simulink model "NEW_MAIN_noDD"  (R2017b)
settings: Solver=ode15s  StartTime=0.0  StopTime=10.0  RelTol=1e-3
values from neighbouring files (symbols this model uses):
  A = eye(16,16)    [full_input_list.m]
  B = zeros(16,1)    [full_input_list.m]
  C = blkdiag(eye(3,3),zeros(3,3),eye(10,10))    [full_input_list.m]
  currentMax_B = [0;0.8;0.2]    [full_input_list.m]
  deltaT = 0.00001    (= 1e-05)    [full_input_list.m]
  epsilon_UD_slew = .01    (= 0.01)    [full_input_list.m]
  epsilon_UD_spinUp = .01    (= 0.01)    [full_input_list.m]
  freq = 80    [full_input_list.m]    (also in initSimulink.m)
  H = C    [full_input_list.m]
  I_UD = [0.032808359, 0.000617048, 0.000049185;      0.000617048, 0.032531573, 0.000060042;      0.000049185, 0.000060042, 0.007799591]    [full_input_list.m]
  kd = 0.5    [full_input_list.m]    (also in initACS.m = 0.01)
  kd_UD_detumble = 6e-3    (= 0.006)    [full_input_list.m]
  kp = 1    [full_input_list.m]    (also in initACS.m = 0.01)
  magMomentMax_B = sat2CoilArea.*sat2n.*currentMax_B    [full_input_list.m]
  omega_cmd_N = 1e-1*[1 1 -.6]'    [full_input_list.m]
  omega_spinUp_MAG = 0.05    [full_input_list.m]
  OpModes = [0 0 0]    [full_input_list.m]
  OpTimes = [0 1 2]    [full_input_list.m]
  q4_cmd_init = [q4_cmd_init(2:4); q4_cmd_init(1)]    [full_input_list.m]
  Q_k = zeros(16,16)    [full_input_list.m]
  R = R_k    [full_input_list.m]
  sat2CoilArea = 0.8*[0.02; 0.02; 0.01]    [full_input_list.m]
  sat2n = [0; 100; 100]    [full_input_list.m]
  sat2Resistance = sat2WireLength.*sat2WireResistivity./sat2WireArea    [full_input_list.m]
  SeperationTime = 30000    [full_input_list.m]
  spinAxis_B = [1 0 0]    [full_input_list.m]
  u_k = zeros(16,1)    [full_input_list.m]
  w_k = zeros(16,1)    [full_input_list.m]
  Z_k = zeros(16,1)    [full_input_list.m]
undefined symbols (not defined in the file or in its folder): B_n, B_N, DiscIntNeverNeededParam, G_igrf, gyro_DCM_BS, H_igrf, I_B, IAU, Kschmidt, mag_variance, Orbit_time, R_mean, r_n, r_N, v_n, v_N
libraries: aerolibutil x53, vrlib x37, simulink x22, SimMainLibrary x14, dspmathops x6, sharedtransform x4, dspinverses x2, dspmtrx3 x1, aerolibtransform2 x1, aerolibgravity2 x1, lib_violet_env x1
(part 1 of 3)
settings Model: Creator=vtroo  LastModifiedBy=vtroo

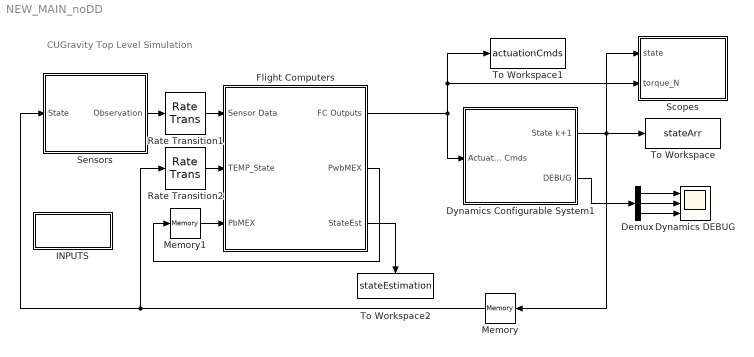
== system NEW_MAIN_noDD ==
  note: CUGravity Top Level Simulation
  Demux : Demux  Outputs=3
  Dynamics Configurable System1 : Subsystem  BlockChoice=Three Link Simscape Model
      link override Extendable Single  Link Simscape /s_teth_init2: PxPositionTargetSpecify=on  PxPositionTargetValue=eps
      link override Single Link Simscape Model/s_teth_init: PxPositionTargetSpecify=on  PxPositionTargetValue=eps  PyPositionTargetSpecify=on  PyPositionTargetValue=eps  PzPositionTargetSpecify=on  PzPositionTargetValue=eps
      link override Single Link Simscape Model/s_teth_init2: PxPositionTargetSpecify=on  PxPositionTargetValue=eps  PyPositionTargetSpecify=on  PyPositionTargetValue=eps  PzPositionTargetSpecify=on  PzPositionTargetValue=eps
      link override Three Link Simscape Model/Attitude Disturbance Model/Aerodynamic Drag/Constant1: Value=G*m_earth
      link override Three Link Simscape Model/Attitude Disturbance Model/Aerodynamic Drag/Gain: Gain=0.5*cd*Ab*p
      link override Three Link Simscape Model/Attitude Disturbance Model/Gravity Gradient/X-Torque/Constant: Value=3*G*m_earth*(I3-I2)
      link override Three Link Simscape Model/Attitude Disturbance Model/Gravity Gradient/Y-Torque/Constant: Value=3*G*m_earth*(I1-I3)
      link override Three Link Simscape Model/Attitude Disturbance Model/Gravity Gradient/Z-Torque/Constant: Value=3*G*m_earth*(I2-I1)
      link override Three Link Simscape Model/Attitude Disturbance Model/Solar Radiation Pressure/Gain: Gain=(flux/c)*Ab*(1+q)
      link override Three Link Simscape Model/Attitude Disturbance Model/Solar Radiation Pressure/Gain1: Gain=(flux/c)*Ab*(1+q)
      link override Three Link Simscape Model/Attitude Disturbance Model/Solar Radiation Pressure/Gain2: Gain=(flux/c)*Ab*(1+q)
      link override Three Link Simscape Model/Bus Selector1: OutputSignals=CenterCube_PWM_cmds,MotorReelRates,BurnCmd,ACSSafeMode
      link override Three Link Simscape Model/CenterSat_6DOF: PxVelocityTargetPriority=Low  PyVelocityTargetPriority=Low  PzVelocityTargetPriority=Low
      link override Three Link Simscape Model/EndSat1_6DOF: PxVelocityTargetPriority=Low  PyVelocityTargetPriority=Low  PzVelocityTargetPriority=Low
      link override Three Link Simscape Model/EndSat2_6DOF: PxVelocityTargetPriority=Low  PyVelocityTargetPriority=Low  PzVelocityTargetPriority=Low
      link override Three Link Simscape Model/Kane Damper 1: SerializedFrames=<Frames><Frame><Id>Frame1</Id><Value><Name>F1</Name><Origin><Source>GeometricFeature</Source><FeatureName>+z surface</FeatureName></Origin><PrimaryAxis><DefinedDirection>+Z</DefinedDirection><Source>ReferenceFrame</Source><SourceDirection>+Z</SourceDirection><FeatureName></FeatureName></PrimaryAxis><SecondaryAxis><DefinedDirection>+X</DefinedDirection><Source>ReferenceFrame</Source><SourceDirection>+X</SourceDirection><FeatureName></FeatureName></SecondaryAxis></Value></Frame></Frames>
      link override Three Link Simscape Model/Kane Damper 2: SerializedFrames=<Frames><Frame><Id>Frame1</Id><Value><Name>F1</Name><Origin><Source>GeometricFeature</Source><FeatureName>-z surface</FeatureName></Origin><PrimaryAxis><DefinedDirection>+Z</DefinedDirection><Source>ReferenceFrame</Source><SourceDirection>+Z</SourceDirection><FeatureName></FeatureName></PrimaryAxis><SecondaryAxis><DefinedDirection>+X</DefinedDirection><Source>ReferenceFrame</Source><SourceDirection>+X</SourceDirection><FeatureName></FeatureName></SecondaryAxis></Value></Frame></Frames>  GeometryShape=Brick  BrickDimensions=[kane_radius kane_radius kane_height]
      link override Three Link Simscape Model/Linear Damper: SpringStiffness=1/(1/linearDamper_k + 1/((pi*teth_radius_actual^2)*teth_modulus/teth_length))
      link override Undeployed Model/Center Sat1: GraphicDiffuseColor=[0.0 0.8 0.8]  GraphicOpacity=.5  SerializedFrames=<Frames><Frame><Id>Frame1</Id><Value><Name>PosZ</Name><Origin><Source>GeometricFeature</Source><FeatureName>+z surface</FeatureName></Origin><PrimaryAxis><DefinedDirection>+Z</DefinedDirection><Source>ReferenceFrame</Source><SourceDirection>+Z</SourceDirection><FeatureName></FeatureName></PrimaryAxis><SecondaryAxis><DefinedDirection>+X</DefinedDirection><Source>ReferenceFrame</Source><SourceDirection>+X</SourceDirection><FeatureName></FeatureName></SecondaryAxis></Value></Frame><Frame><Id>Frame2</Id><Value><Name>NegZ</Name><Origin><Source>GeometricFeature</Source><FeatureName>-z surface</FeatureName></Origin><PrimaryAxis><DefinedDirection>+Z</DefinedDirection><Source>ReferenceFrame</Source><SourceDirection>+Z</SourceDirection><FeatureName></FeatureName></PrimaryAxis><SecondaryAxis><DefinedDirection>+X</DefinedDirection><Source>ReferenceFrame</Source><SourceDirection>+X</SourceDirection><FeatureName></FeatureName></SecondaryAxis></Value></Frame><Frame><Id>Frame7</Id><Value><Name>PosX</Name><Origin><Source>GeometricFeature</Source><FeatureName>+x surface</FeatureName></Origin><PrimaryAxis><DefinedDirection>+Z</DefinedDirection><Source>ReferenceFrame</Source><SourceDirection>+Z</SourceDirection><FeatureName></FeatureName></PrimaryAxis><SecondaryAxis><DefinedDirection>+X</DefinedDirection><Source>ReferenceFrame</Source><SourceDirection>+X</SourceDirection><FeatureName></FeatureName></SecondaryAxis></Value></Frame><Frame><Id>Frame8</Id><Value><Name>COM</Name><Origin><Source>CenterOfMassFrame</Source><FeatureName></FeatureName></Origin><PrimaryAxis><DefinedDirection>+Z</DefinedDirection><Source>ReferenceFrame</Source><SourceDirection>+Z</SourceDirection><FeatureName></FeatureName></PrimaryAxis><SecondaryAxis><DefinedDirection>+X</DefinedDirection><Source>ReferenceFrame</Source><SourceDirection>+X</SourceDirection><FeatureName></FeatureName></SecondaryAxis></Value></Frame></Frames>
      link override Undeployed Model/EndSat3: GraphicOpacity=.5  GraphicDiffuseColor=[1.0 0.0 0.0]
      link override Undeployed Model/EndSat4: GraphicOpacity=.5  GraphicDiffuseColor=[1.0 0.0 0.0]
      settings: AttributesFormatString=%<BlockChoice>  TemplateBlock=SimMainLibrary/Dynamics Configurable System  MemberBlocks="Extendable Single  Link Simscape ,Single Link Simscape Model,Three Link Simscape Model,Undeployed Model"
  Dynamics DEBUG : Scope  NumInputPorts=3
  Flight Computers : Subsystem  mask(Flight Computers){}
      mask help:
      | The flight computers read in the measured state from the sensor block and the previous PowerBoard commands and state (inputs). The ground commands are also inputs to receive potential command override. This information is then passed through the Kalman filter to estimate the state and remove sensor noise, and sent through a controller which determines the operation mode, updated PowerBoard Status, and actuator commands. These outputs govern the operation of the satellite and deterine the trajectory it will follow in the future steps.
      |
      | NOTE: Currently the UKF is not complete, and for that reason the input state read into the controller is simply the exact state outputted from the dynamics block. That is, the sensor block is going unused because there is no way to currently remove sensor noise (UKF). Once the UKF is completed, the sensor measurements must be used for the controller inputs to simulate a more realistic environment.
  INPUTS : Subsystem
  Memory : Memory  InheritSampleTime=on
  Memory1 : Memory  InheritSampleTime=on
  Rate Transition1 : RateTransition  OutPortSampleTime=1/freq
  Rate Transition2 : RateTransition  OutPortSampleTime=1/freq
  Scopes : Subsystem
  Sensors : Subsystem  mask(State Estimation){}
      mask help:
      | Current Function:
      | This block uses the plant model calculated state (input) and adds sensor noise to the system to calculate the estimated state (output) that is measured and fed into the flight computer. The middle satellite has a more extensive set of calculations required to complete the state estimation, than do the end satellites. All three satellites compute the accelerometer, magnetometer, angular velocity, and sun sensor vector measurements. The middle satellite performs additional calculations to accurately measure simulation time and inertial position of the center of mass.
      |
      | Future Tasks:
      | 1. Make sure that q1_BN is quaternion of B relative to N, otherwise rotation may be in the wrong direction.
      | 2. Need to test the calculation to find the sun vector in the B frame.
  To Workspace : ToWorkspace  VariableName=stateArr  SaveFormat=Timeseries  SampleTime=-1
  To Workspace1 : ToWorkspace  VariableName=actuationCmds  SaveFormat=Timeseries  SampleTime=-1
  To Workspace2 : ToWorkspace  VariableName=stateEstimation  SaveFormat=Timeseries  SampleTime=-1
  wires:
  Rate Transition1/1 -> Flight Computers/1(Sensor Data)
  Flight Computers/1(FC Outputs) -> To Workspace1/1, Scopes/2(torque_N), Dynamics Configurable System1/1(Actuation Cmds)
  Demux/3 -> Dynamics DEBUG/3
  Rate Transition2/1 -> Flight Computers/2(TEMP_State)
  Demux/2 -> Dynamics DEBUG/2
  Flight Computers/2(PwbMEX) -> Memory1/1
  Dynamics Configurable System1/1(State k+1) -> Scopes/1(state), Memory/1, To Workspace/1
  Sensors/1(Observation) -> Rate Transition1/1
  Flight Computers/3(StateEst) -> To Workspace2/1
  Demux/1 -> Dynamics DEBUG/1
  Memory/1 -> Sensors/1(State), Rate Transition2/1
  Memory1/1 -> Flight Computers/3(PbMEX)
  Dynamics Configurable System1/2(DEBUG) -> Demux/1

== system NEW_MAIN_noDD/Dynamics Configurable System1 ==
  Actuation Cmds : Inport
  Three Link Simscape Model : SimMainLibrary/Three Link Simscape Model
      settings: SourceProductName=CUGravity Library
  State k+1 : Outport
  DEBUG : Outport  Port=2
  wires:
  Actuation Cmds/1 -> Three Link Simscape Model/1
  Three Link Simscape Model/1 -> State k+1/1
  Three Link Simscape Model/2 -> DEBUG/1

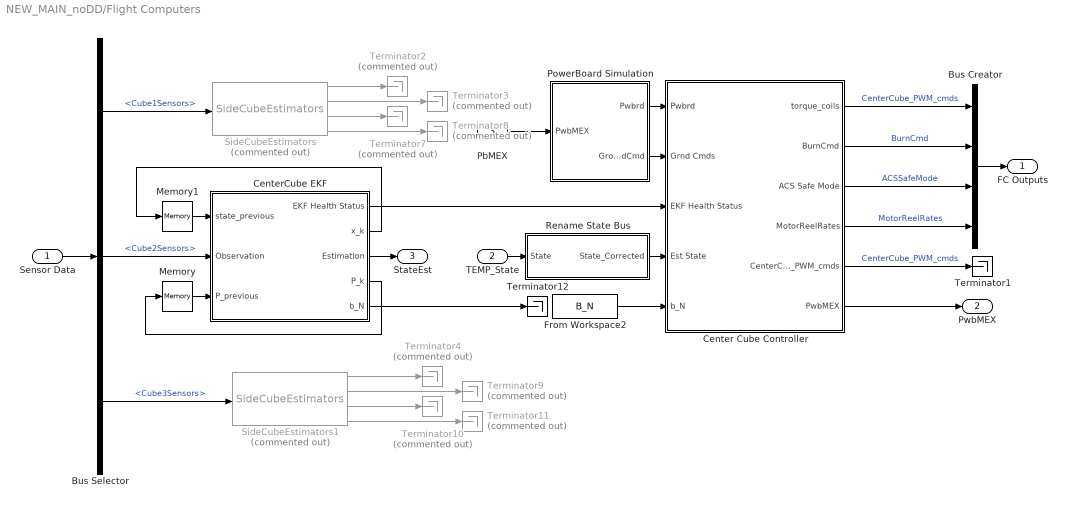
== system NEW_MAIN_noDD/Flight Computers ==
  Sensor Data : Inport
  TEMP_State : Inport  Port=2
  PbMEX : Inport  Port=3
  Bus Creator : BusCreator  Inputs=4
  Bus Selector : BusSelector  OutputSignals=Cube1Sensors,Cube2Sensors,Cube3Sensors
  Center Cube Controller : Subsystem
  CenterCube EKF : Subsystem
  From Workspace2 : FromWorkspace  VariableName=B_N  SampleTime=1/freq
  Memory : Memory
  Memory1 : Memory
  PowerBoard Simulation : Subsystem  mask(Command and Operation){}
      mask help:
      | Current Function:
      | Determines commands based on the PowerBoard as well as messages received from ground control. It also has the status of the sensor and torque actuator signals to feed into the state machine.
      |
      | Future Tasks:
      | Currently the ground commands and PowerBoard commands are the same, so there should probably be a way to allow manual override for ground control purposes.
  Rename State Bus : Subsystem  mask(State Correction){}
      mask help:
      | Current Function:
      | This block is only a PLACEHOLDER for the time being: until the UKF is complete, this block shall be used to feed in the EXACT state (dynamics) to the controller. However, the memory block causes issues with the initial condition for the quaternions, so this block performs a correction such that the norm of the quaternion is always unity (one). Additionally, the connections within the bus must be named as estimated values to be compatible with calculations performed within the controller.
      |
      | Future Task:
      | Complete UKF. Delete this subsystem. Feed the Estimated state output from the UKF into the controller (instead of this output).
  SideCubeEstimators : SimMainLibrary/SideCubeEstimators  Commented=on
      settings: SourceProductName=CUGravity Library
  SideCubeEstimators1 : SimMainLibrary/SideCubeEstimators  Commented=on
      settings: SourceProductName=CUGravity Library
  Terminator1 : Terminator
  Terminator{2..4,7..11} (8 alike) : Terminator  Commented=on
  Terminator12 : Terminator
  FC Outputs : Outport
  PwbMEX : Outport  Port=2
  StateEst : Outport  Port=3
  wires:
  Sensor Data/1 -> Bus Selector/1
  Bus Selector/1 -> SideCubeEstimators/1  "<Cube1Sensors>"
  Bus Selector/2 -> CenterCube EKF/2(Observation)  "<Cube2Sensors>"
  Bus Selector/3 -> SideCubeEstimators1/1  "<Cube3Sensors>"
  SideCubeEstimators/1 -> Terminator2/1
  Bus Creator/1 -> FC Outputs/1
  Center Cube Controller/2(BurnCmd) -> Bus Creator/2  "BurnCmd"
  CenterCube EKF/1(EKF Health Status) -> Center Cube Controller/3("EKF Health Status ")
  Center Cube Controller/6(PwbMEX) -> PwbMEX/1
  CenterCube EKF/3(Estimation) -> StateEst/1
  Center Cube Controller/5(CenterCube_PWM_cmds) -> Terminator1/1  "CenterCube_PWM_cmds"
  SideCubeEstimators/2 -> Terminator3/1
  CenterCube EKF/2(x_k) -> Memory1/1
  CenterCube EKF/4(P_k) -> Memory/1
  SideCubeEstimators/3 -> Terminator7/1
  SideCubeEstimators/4 -> Terminator8/1
  SideCubeEstimators1/1 -> Terminator4/1
  SideCubeEstimators1/2 -> Terminator9/1
  SideCubeEstimators1/3 -> Terminator10/1
  SideCubeEstimators1/4 -> Terminator11/1
  Center Cube Controller/3(ACS Safe Mode) -> Bus Creator/3  "ACSSafeMode"
  Center Cube Controller/4(MotorReelRates) -> Bus Creator/4  "MotorReelRates"
  Center Cube Controller/1(torque_coils) -> Bus Creator/1  "CenterCube_PWM_cmds"
  From Workspace2/1 -> Center Cube Controller/5(b_N)
  CenterCube EKF/5(b_N) -> Terminator12/1
  TEMP_State/1 -> Rename State Bus/1(State)
  PbMEX/1 -> PowerBoard Simulation/1(PwbMEX)
  PowerBoard Simulation/1(Pwbrd) -> Center Cube Controller/1(Pwbrd)
  PowerBoard Simulation/2(GroundCmd) -> Center Cube Controller/2(Grnd Cmds)
  Rename State Bus/1(State_Corrected) -> Center Cube Controller/4(Est State)
  Memory/1 -> CenterCube EKF/3(P_previous)
  Memory1/1 -> CenterCube EKF/1(state_previous)

== system NEW_MAIN_noDD/INPUTS ==
  Chart : Stateflow chart  Commented=on  TreatAsAtomicUnit=on
  Clock : Clock  Commented=on
  Constant : Constant  Commented=on  Value=Orbit_time
  Constant1 : Constant  Commented=on  Value=r_n
  Constant2 : Constant  Commented=on  Value=v_n
  Constant3 : Constant  Commented=on  Value=B_n
  Constant4 : Constant  Commented=on  Value=Orbit_time(1)
  Constant5 : Constant  Commented=on  Value=ones(1,length(Orbit_time))
  Constant6 : Constant  Commented=on  Value=r_N
  Constant7 : Constant  Commented=on  Value=v_N
  Constant8 : Constant  Commented=on  Value=B_N
  From Workspace : FromWorkspace  Commented=on  VariableName=r_N  SampleTime=1/freq
  From Workspace1 : FromWorkspace  Commented=on  VariableName=v_N  SampleTime=1/freq
  From Workspace2 : FromWorkspace  Commented=on  VariableName=B_N  SampleTime=1/freq
  Product : Product  Commented=on
  Sum : Sum  Commented=on  Inputs=|+-
  Terminator : Terminator  Commented=on
  Terminator1 : Terminator  Commented=on
  Terminator2 : Terminator  Commented=on
  wires:
  Clock/1 -> Product/2
  Constant/1 -> Sum/1
  Constant1/1 -> Chart/3(r_N)
  Constant2/1 -> Chart/4(v_N)
  Constant3/1 -> Chart/5(B_N)
  Sum/1 -> Chart/2(T)
  Constant4/1 -> Sum/2
  Product/1 -> Chart/1(t)
  Constant5/1 -> Product/1
  Chart/1(r) -> Terminator/1
  Chart/2(v) -> Terminator1/1
  Chart/3(B) -> Terminator2/1

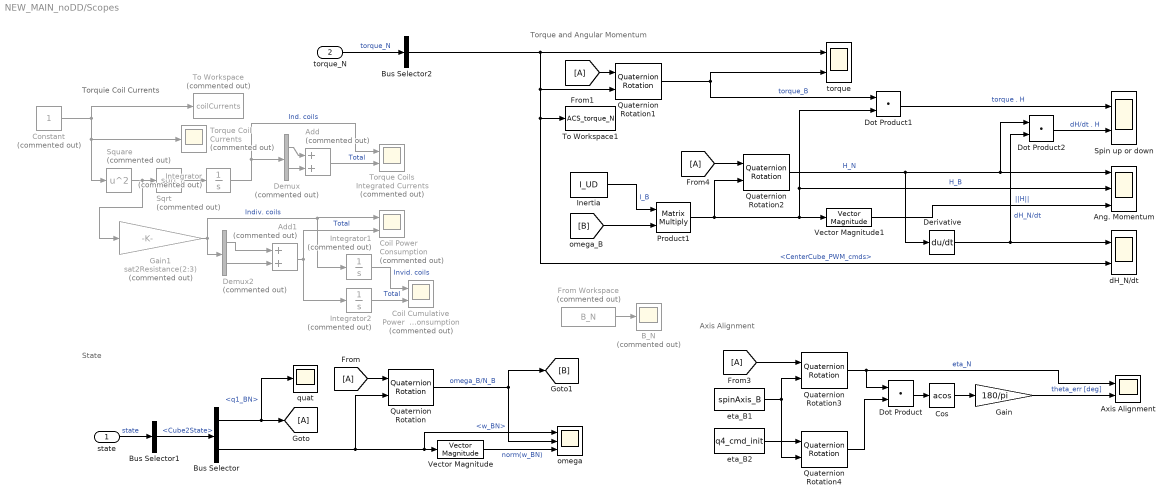
== system NEW_MAIN_noDD/Scopes ==
  note: State
  note: Torque and Angular Momentum
  note: Axis Alignment
  note: Torquie Coil Currents
  state : Inport
  torque_N : Inport  Port=2
  Add : Sum  Commented=on
  Add1 : Sum  Commented=on
  Ang. Momentum : Scope  NumInputPorts=3
  Axis Alignment : Scope  NumInputPorts=2
  B_N : Scope  Commented=on
  Bus Selector : BusSelector  OutputSignals=q1_BN,w_BN
  Bus Selector1 : BusSelector  OutputSignals=Cube2State
  Bus Selector2 : BusSelector  OutputSignals=CenterCube_PWM_cmds
  Coil Cumulative Power  Consumption : Scope  Commented=on  NumInputPorts=2
  Coil Power Consumption : Scope  Commented=on  NumInputPorts=2
  Constant : Constant  Commented=on
  Cos : Trigonometry  Operator=acos  OutputSignalType=real
  Demux : Demux  Commented=on  Outputs=2
  Demux2 : Demux  Commented=on  Outputs=2
  Derivative : Derivative
  Dot Product : DotProduct  InputSameDT=on  OutDataTypeStr=Inherit: Inherit via internal rule
  Dot Product1 : DotProduct  InputSameDT=on  OutDataTypeStr=Inherit: Inherit via internal rule
  Dot Product2 : DotProduct  InputSameDT=on  OutDataTypeStr=Inherit: Inherit via internal rule
  From Workspace : FromWorkspace  Commented=on  VariableName=B_N  SampleTime=0
  Gain : Gain  Gain=180/pi
  Gain1 : Gain  Commented=on  Gain=sat2Resistance(2:3)
  Inertia : Constant  Value=I_UD
  Integrator : Integrator  Commented=on
  Integrator1 : Integrator  Commented=on
  Integrator2 : Integrator  Commented=on
  Product1 : Product  Multiplication=Matrix(*)
  Quaternion Rotation{,1..4} (5 alike) : aerolibutil/Quaternion Rotation
  Spin up or down : Scope  NumInputPorts=2
  Sqrt : Sqrt  Commented=on  SaturateOnIntegerOverflow=on
  Square : Math  Commented=on  Operator=square  RndMeth=Zero  SaturateOnIntegerOverflow=on
  To Workspace : ToWorkspace  Commented=on  VariableName=coilCurrents  SaveFormat=Timeseries  SampleTime=-1
  To Workspace1 : ToWorkspace  VariableName=ACS_torque_N  SaveFormat=Timeseries  SampleTime=-1
  Torque Coil Currents : Scope  Commented=on
  Torque Coils Integrated Currents : Scope  Commented=on  NumInputPorts=2
  Vector Magnitude : SimMainLibrary/Vector Magnitude
      settings: SourceProductName=CUGravity Library
  Vector Magnitude1 : SimMainLibrary/Vector Magnitude
      settings: SourceProductName=CUGravity Library
  dH_N/dt : Scope  NumInputPorts=2
  eta_B1 : Constant  Value=spinAxis_B
  eta_B2 : Constant  Value=q4_cmd_init
  omega : Scope  NumInputPorts=3
  quat : Scope
  torque : Scope  NumInputPorts=2
  wires:
  Constant/1 -> Square/1, Torque Coil Currents/1, To Workspace/1
  Integrator/1 -> Demux/1, Torque Coils Integrated Currents/1  "Ind. coils"
  Cos/1 -> Gain/1
  Quaternion Rotation3/1 -> Dot Product/1, Axis Alignment/1  "eta_N"
  eta_B1/1 -> Quaternion Rotation4/2, Quaternion Rotation3/2
  Quaternion Rotation4/1 -> Dot Product/2
  eta_B2/1 -> Quaternion Rotation4/1
  [A] -> Quaternion Rotation3/1
  Dot Product/1 -> Cos/1
  Gain/1 -> Axis Alignment/2  "theta_err [deg]"
  Bus Selector2/1 -> dH_N/dt/2, To Workspace1/1, Quaternion Rotation1/2, torque/1  "<CenterCube_PWM_cmds>"
  [B] -> Product1/2
  Dot Product1/1 -> Spin up or down/1  "torque . H"
  Derivative/1 -> Dot Product2/2, dH_N/dt/1  "dH_N/dt"
  Vector Magnitude1/1 -> Ang. Momentum/3  "||H||"
  [A] -> Quaternion Rotation1/1
  Product1/1 -> Vector Magnitude1/1, Ang. Momentum/2, Dot Product1/2, Quaternion Rotation2/2  "H_B"
  Inertia/1 -> Product1/1  "I_B"
  Quaternion Rotation1/1 -> Dot Product1/1, torque/2  "torque_B"
  [A] -> Quaternion Rotation2/1
  Quaternion Rotation2/1 -> Derivative/1, Dot Product2/1, Ang. Momentum/1  "H_N"
  Bus Selector/2 -> Quaternion Rotation/2, omega/1, Vector Magnitude/1  "<w_BN>"
  Quaternion Rotation/1 -> omega/2, [B]  "omega_B/N_B"
  Bus Selector/1 -> quat/1, [A]  "<q1_BN>"
  Vector Magnitude/1 -> omega/3  "norm(w_BN)"
  Square/1 -> Gain1/1, Sqrt/1
  Sqrt/1 -> Integrator/1
  Demux/1 -> Add/1
  Demux/2 -> Add/2
  Add/1 -> Torque Coils Integrated Currents/2  "Total"
  Gain1/1 -> Integrator1/1, Coil Power Consumption/1, Demux2/1  "Indiv. coils"
  Demux2/1 -> Add1/1
  Demux2/2 -> Add1/2
  Add1/1 -> Integrator2/1, Coil Power Consumption/2  "Total"
  Integrator1/1 -> Coil Cumulative Power  Consumption/1  "Invid. coils"
  Integrator2/1 -> Coil Cumulative Power  Consumption/2  "Total"
  state/1 -> Bus Selector1/1  "state"
  Bus Selector1/1 -> Bus Selector/1  "<Cube2State>"
  torque_N/1 -> Bus Selector2/1  "torque_N"
  Dot Product2/1 -> Spin up or down/2  "dH/dt . H"
  From Workspace/1 -> B_N/1
  [A] -> Quaternion Rotation/1

== system NEW_MAIN_noDD/Sensors ==
  note: Sensor Blocks:
      | -The SideCube blocks are library blocks to because they are the same
      | -Center Cube is not
  State : Inport
  Bus Creator1 : BusCreator  Inputs=3
  Bus Selector1 : BusSelector  OutputSignals=Cube1State,Cube2State,Cube3State
  Center Cube Sensors : Subsystem
  EndSat Sensor1 : Subsystem
  EndSat Sensor2 : Subsystem
  From Workspace2 : FromWorkspace  VariableName=B_N  SampleTime=1/freq
  Observation : Outport
  wires:
  Bus Creator1/1 -> Observation/1
  Bus Selector1/1 -> EndSat Sensor1/1(State)  "<Cube1State>"
  EndSat Sensor1/1(Sensors) -> Bus Creator1/1  "Cube1Sensors"
  EndSat Sensor2/1(Sensors) -> Bus Creator1/3  "Cube3Sensors"
  Center Cube Sensors/1(Sensors) -> Bus Creator1/2  "Cube2Sensors"
  Bus Selector1/2 -> Center Cube Sensors/1(State)  "<Cube2State>"
  Bus Selector1/3 -> EndSat Sensor2/1(State)  "<Cube3State>"
  State/1 -> Bus Selector1/1
  From Workspace2/1 -> EndSat Sensor2/2(B_N), Center Cube Sensors/2(B_N), EndSat Sensor1/2(B_N)

== system NEW_MAIN_noDD/Flight Computers/Center Cube Controller ==
  Pwbrd : Inport
  Grnd Cmds : Inport  Port=2
  "EKF Health Status " : Inport  Port=3
  Est State : Inport  Port=4
  b_N : Inport  Port=5
  Bus Selector : BusSelector  OutputSignals=w_BN_est
  Bus Selector1 : BusSelector  OutputSignals=q_BN_est
  Display : Display
  Memory : Memory  InheritSampleTime=on
  Motor Controller Scope : Scope
  SafeMode : Subsystem
  "Sequential Motor Controller " : SimMainLibrary/Sequential Motor Controller
      settings: SourceProductName=CUGravity Library
  Torque Coil Management : Subsystem  mask(Navigation and Torque Coil Management Block){}
      mask help:
      | This block takes in data from the actions/guidance block as to the current attitude of the spacecraft, the desired attitude of the spacecraft, and the required torque and outputs the current necessary to be applied to the torque coils as well as the torque currently being applied by the torque coils.
      |
      | This block takes in the needed torque to perform an attitude changing maneuver, the current position, and the body reference frame. It outputs the current needed in each coil and the resulting output torque of each coil.
      |
      | Equations used:
      | 1. torque_B = mu_B x B_B
      | 2. B_B = Q_B/N x b_N
      | 3. Mu = I*n*A_B
      |
      | Author: Aaron Sandoval
  torque_coils : Outport
  BurnCmd : Outport  Port=2
  ACS Safe Mode : Outport  Port=3
  MotorReelRates : Outport  Port=4
  CenterCube_PWM_cmds : Outport  Port=5
  PwbMEX : Outport  Port=6
  wires:
  Memory/1 -> SafeMode/2(Safe Mode In)
  SafeMode/2(SafedSeperationBurn) -> BurnCmd/1
  Est State/1 -> SafeMode/5(EstState)
  SafeMode/1(SafedOpMode) -> "Sequential Motor Controller "/2
  Grnd Cmds/1 -> SafeMode/1(GrndCmds)
  "EKF Health Status "/1 -> SafeMode/4("EKFhs ")
  Pwbrd/1 -> SafeMode/3(Pwbrd)
  Torque Coil Management/1(torque_coils) -> torque_coils/1
  SafeMode/5(Safed Att. State) -> Bus Selector1/1, Bus Selector/1
  SafeMode/6(Safe Mode Out) -> Memory/1, Display/1, ACS Safe Mode/1
  SafeMode/3(PwbMEX) -> PwbMEX/1
  "Sequential Motor Controller "/1 -> MotorReelRates/1
  "Sequential Motor Controller "/2 -> Motor Controller Scope/1
  b_N/1 -> [B_N], SafeMode/6(B_N)
  Bus Selector/1 -> "Sequential Motor Controller "/1  "<w_BN_est>"
  [B_N] -> Torque Coil Management/1(B_N)
  SafeMode/4(T_N) -> Torque Coil Management/2(torque_cmd_N)
  Bus Selector1/1 -> Torque Coil Management/3(q)  "<q_BN_est>"
  Torque Coil Management/2(CenterCube_PWM_cmds) -> CenterCube_PWM_cmds/1

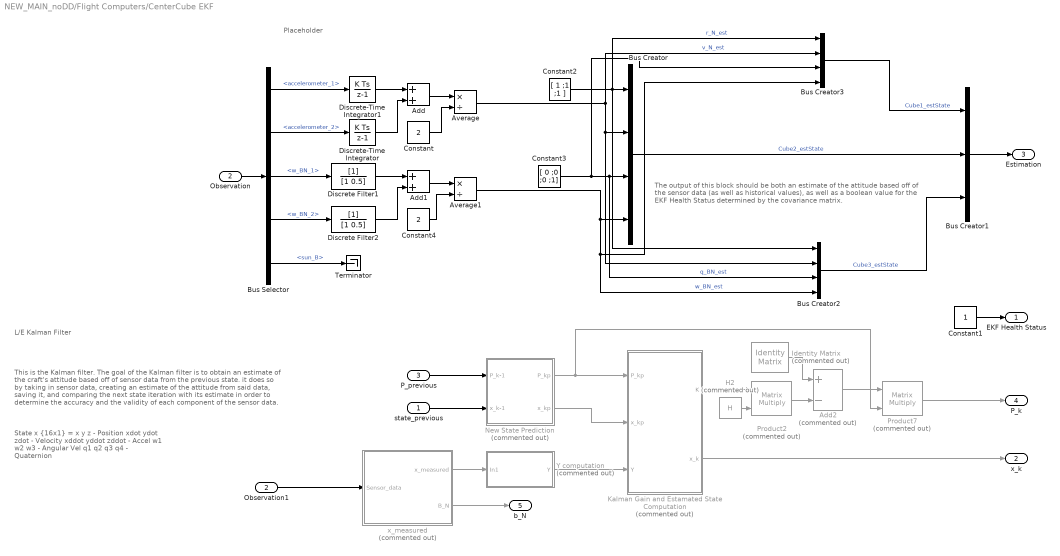
== system NEW_MAIN_noDD/Flight Computers/CenterCube EKF ==
  note: The output of this block should be both an estimate of the attitude based off of the sensor data (as well as historical values), as well as a boolean value for the EKF Health Status determined by the covariance matrix.
  note: Placeholder
  note: This is the Kalman filter. The goal of the Kalman filter is to obtain an estimate of the craft's attitude based off of sensor data from the previous state. it does so by taking in sensor data, creating an estimate of the attitude from said data, saving it, and comparing the next state iteration with its estimate in order to determine the accuracy and the validity of each component of the sensor data.
  note: L/E Kalman Filter
  note: State x {16x1} =
      | x y z - Position
      | xdot ydot zdot - Velocity
      | xddot yddot zddot - Accel
      | w1 w2 w3 - Angular Vel
      | q1 q2 q3 q4 - Quaternion
  state_previous : Inport
  Observation : Inport  Port=2
  P_previous : Inport  Port=3
  Add : Sum
  Add1 : Sum
  Add2 : Sum  Commented=on  Inputs=+-
  Average : Product  Inputs=*/
  Average1 : Product  Inputs=*/
  Bus Creator : BusCreator  Inputs=4
  Bus Creator1 : BusCreator  Inputs=3
  Bus Creator2 : BusCreator  Inputs=4
  Bus Creator3 : BusCreator  Inputs=4
  Bus Selector : BusSelector  OutputSignals=accelerometer_1,accelerometer_2,w_BN_1,w_BN_2,sun_B
  Constant : Constant  Value=2
  Constant1 : Constant
  Constant2 : Constant  Value=[ 1 ;1 ;1 ]
  Constant3 : Constant  Value=[ 0 ;0 ;0 ;1]
  Constant4 : Constant  Value=2
  Discrete Filter1 : DiscreteFilter
  Discrete Filter2 : DiscreteFilter
  Discrete-Time Integrator : DiscreteIntegrator  InitialConditionSetting=State (most efficient)  SampleTime=-1  ICPrevOutput=DiscIntNeverNeededParam  ICPrevScaledInput=DiscIntNeverNeededParam
  Discrete-Time Integrator1 : DiscreteIntegrator  InitialConditionSetting=State (most efficient)  SampleTime=-1  ICPrevOutput=DiscIntNeverNeededParam  ICPrevScaledInput=DiscIntNeverNeededParam
  H2 : Constant  Commented=on  Value=H
  Identity Matrix : dspmtrx3/Identity Matrix  Commented=on  Inherit=off  N=16  Ts=1  dataType=double  isSigned=on  wordLen=16  udDataType=sfix(16)  fracBitsMode=Best precision  numFracBits=15  OutDataTypeStr=double  LastOutDataTypeStr=double
      settings: SourceProductName=DSP System Toolbox
  Kalman Gain and Estamated State Computation : Subsystem  Commented=on
  "New State Prediction " : Subsystem  Commented=on
  Observation1 : InportShadow  Port=2
  Product2 : Product  Commented=on  Multiplication=Matrix(*)
  Product7 : Product  Commented=on  Multiplication=Matrix(*)
  Terminator : Terminator
  Y computation : Subsystem  Commented=on
  x_measured : Subsystem  Commented=on
  EKF Health Status : Outport
  x_k : Outport  Port=2
  Estimation : Outport  Port=3
  P_k : Outport  Port=4
  b_N : Outport  Port=5
  wires:
  Bus Selector/2 -> Discrete-Time Integrator/1  "<accelerometer_2>"
  Discrete-Time Integrator/1 -> Add/2
  Bus Selector/4 -> Discrete Filter2/1  "<w_BN_2>"
  Add/1 -> Average/1
  Constant/1 -> Average/2
  Average/1 -> Bus Creator2/2, Bus Creator/2, Bus Creator3/2  "v_N_est"
  Bus Selector/1 -> Discrete-Time Integrator1/1  "<accelerometer_1>"
  Bus Selector/3 -> Discrete Filter1/1  "<w_BN_1>"
  Observation/1 -> Bus Selector/1
  Bus Creator/1 -> Bus Creator1/2  "Cube2_estState"
  Constant3/1 -> Bus Creator3/3, Bus Creator2/3, Bus Creator/3  "q_BN_est"
  Constant2/1 -> Bus Creator3/1, Bus Creator2/1, Bus Creator/1  "r_N_est"
  Average1/1 -> Bus Creator2/4, Bus Creator3/4, Bus Creator/4  "w_BN_est"
  Bus Selector/5 -> Terminator/1  "<sun_B>"
  Discrete-Time Integrator1/1 -> Add/1
  Discrete Filter2/1 -> Add1/2
  Add1/1 -> Average1/1
  Constant4/1 -> Average1/2
  Discrete Filter1/1 -> Add1/1
  Bus Creator1/1 -> Estimation/1
  Bus Creator3/1 -> Bus Creator1/1  "Cube1_estState"
  Bus Creator2/1 -> Bus Creator1/3  "Cube3_estState"
  Constant1/1 -> EKF Health Status/1
  P_previous/1 -> "New State Prediction "/1(P_k-1)
  state_previous/1 -> "New State Prediction "/2(x_k-1)
  "New State Prediction "/1(P_kp) -> Product7/2, Kalman Gain and Estamated State Computation/1(P_kp)
  Kalman Gain and Estamated State Computation/2(x_k) -> x_k/1
  Identity Matrix/1 -> Add2/1
  H2/1 -> Product2/2
  Product2/1 -> Add2/2
  Add2/1 -> Product7/1
  Product7/1 -> P_k/1
  Kalman Gain and Estamated State Computation/1(K) -> Product2/1
  "New State Prediction "/2("x_kp  ") -> Kalman Gain and Estamated State Computation/2(x_kp)
  Y computation/1(Y) -> Kalman Gain and Estamated State Computation/3(Y)
  x_measured/1(x_measured) -> Y computation/1(In1)
  x_measured/2(B_N) -> b_N/1
  Observation1/1 -> x_measured/1(Sensor_data)

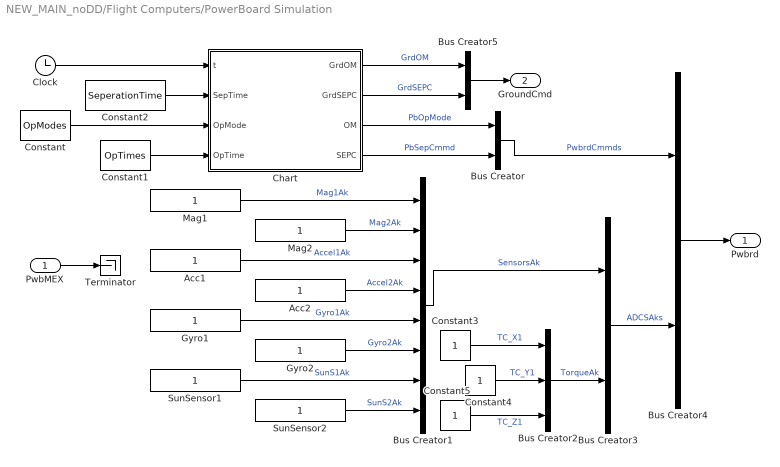
== system NEW_MAIN_noDD/Flight Computers/PowerBoard Simulation ==
  PwbMEX : Inport
  Acc1 : Constant
  Acc2 : Constant
  Bus Creator{,3..5} (4 alike) : BusCreator  Inputs=2
  Bus Creator1 : BusCreator  Inputs=8
  Bus Creator2 : BusCreator  Inputs=3
  Chart : Stateflow chart  TreatAsAtomicUnit=on
  Clock : Clock
  Constant : Constant  Value=OpModes
  Constant1 : Constant  Value=OpTimes
  Constant2 : Constant  Value=SeperationTime
  Constant3 : Constant
  Constant4 : Constant
  Constant5 : Constant
  Gyro1 : Constant
  Gyro2 : Constant
  Mag1 : Constant
  Mag2 : Constant
  SunSensor1 : Constant
  SunSensor2 : Constant
  Terminator : Terminator
  Pwbrd : Outport
  GroundCmd : Outport  Port=2
  wires:
  Constant/1 -> Chart/3(OpMode)
  Constant1/1 -> Chart/4(OpTime)
  Constant2/1 -> Chart/2(SepTime)
  Chart/4(SEPC) -> Bus Creator/2  "PbSepCmmd"
  Bus Creator/1 -> Bus Creator4/1  "PwbrdCmmds"
  Acc2/1 -> Bus Creator1/4  "Accel2Ak"
  Acc1/1 -> Bus Creator1/3  "Accel1Ak"
  Mag1/1 -> Bus Creator1/1  "Mag1Ak"
  Mag2/1 -> Bus Creator1/2  "Mag2Ak"
  Bus Creator1/1 -> Bus Creator3/1  "SensorsAk"
  Constant3/1 -> Bus Creator2/1  "TC_X1"
  Constant4/1 -> Bus Creator2/2  "TC_Y1"
  Constant5/1 -> Bus Creator2/3  "TC_Z1"
  Bus Creator2/1 -> Bus Creator3/2  "TorqueAk"
  Bus Creator3/1 -> Bus Creator4/2  "ADCSAks"
  Bus Creator4/1 -> Pwbrd/1
  Gyro1/1 -> Bus Creator1/5  "Gyro1Ak"
  Gyro2/1 -> Bus Creator1/6  "Gyro2Ak"
  SunSensor1/1 -> Bus Creator1/7  "SunS1Ak"
  SunSensor2/1 -> Bus Creator1/8  "SunS2Ak"
  PwbMEX/1 -> Terminator/1
  Clock/1 -> Chart/1(t)
  Chart/3(OM) -> Bus Creator/1  "PbOpMode"
  Chart/1(GrdOM) -> Bus Creator5/1  "GrdOM"
  Chart/2(GrdSEPC) -> Bus Creator5/2  "GrdSEPC"
  Bus Creator5/1 -> GroundCmd/1

== system NEW_MAIN_noDD/Flight Computers/Rename State Bus ==
  State : Inport
  Bus Creator : BusCreator  Inputs=4
  Bus Creator1 : BusCreator  Inputs=3
  Bus Creator2 : BusCreator  Inputs=4
  Bus Creator3 : BusCreator  Inputs=4
  Bus Selector : BusSelector  OutputSignals=r_N,v_N,q1_BN,w_BN
  Bus Selector1 : BusSelector  OutputSignals=Cube1State,Cube2State,Cube3State
  Bus Selector2 : BusSelector  OutputSignals=r_N,v_N,q1_BN,w_BN
  Bus Selector3 : BusSelector  OutputSignals=r_N,v_N,q1_BN,w_BN
  Constant : Constant
  Constant1 : Constant  Value=2
  Constant3 : Constant  Value=3
  Gain{,1..8} (9 alike) : Gain
  Quat IC Override : SimMainLibrary/Quat IC Override
      settings: SourceProductName=CUGravity Library
  Quat IC Override1 : SimMainLibrary/Quat IC Override
      settings: SourceProductName=CUGravity Library
  Quat IC Override3 : SimMainLibrary/Quat IC Override
      settings: SourceProductName=CUGravity Library
  State_Corrected : Outport
  wires:
  State/1 -> Bus Selector1/1
  Bus Selector1/2 -> Bus Selector2/1  "<Cube2State>"
  Bus Selector1/1 -> Bus Selector/1  "<Cube1State>"
  Bus Creator1/1 -> State_Corrected/1
  Bus Selector1/3 -> Bus Selector3/1  "<Cube3State>"
  Bus Selector/1 -> Gain/1  "<r_N>"
  Bus Selector/2 -> Gain1/1  "<v_N>"
  Bus Creator/1 -> Bus Creator1/1  "Cube1_estState"
  Bus Selector2/2 -> Gain5/1  "<v_N>"
  Bus Selector2/1 -> Gain4/1  "<r_N>"
  Bus Creator2/1 -> Bus Creator1/2  "Cube2_estState"
  Bus Creator3/1 -> Bus Creator1/3  "Cube3_estState"
  Gain4/1 -> Bus Creator2/1  "r_N_est"
  Gain5/1 -> Bus Creator2/2  "v_N_est"
  Quat IC Override1/1 -> Bus Creator2/3  "q_BN_est"
  Gain7/1 -> Bus Creator2/4  "w_BN_est"
  Constant/1 -> Quat IC Override/2
  Bus Selector2/3 -> Quat IC Override1/1  "<q1_BN>"
  Constant1/1 -> Quat IC Override1/2
  Bus Selector/3 -> Quat IC Override/1  "<q1_BN>"
  Bus Selector/4 -> Gain3/1  "<w_BN>"
  Bus Selector2/4 -> Gain7/1  "<w_BN>"
  Bus Selector3/3 -> Quat IC Override3/1  "<q1_BN>"
  Gain6/1 -> Bus Creator3/2  "v_N_est"
  Gain2/1 -> Bus Creator3/1  "r_N_est"
  Bus Selector3/2 -> Gain6/1  "<v_N>"
  Bus Selector3/4 -> Gain8/1  "<w_BN>"
  Gain8/1 -> Bus Creator3/4  "w_BN_est"
  Constant3/1 -> Quat IC Override3/2
  Quat IC Override3/1 -> Bus Creator3/3  "q_BN_est"
  Bus Selector3/1 -> Gain2/1  "<r_N>"
  Gain3/1 -> Bus Creator/4  "w_BN_est"
  Gain1/1 -> Bus Creator/2  "v_N_est"
  Gain/1 -> Bus Creator/1  "r_N_est"
  Quat IC Override/1 -> Bus Creator/3  "q_BN_est"

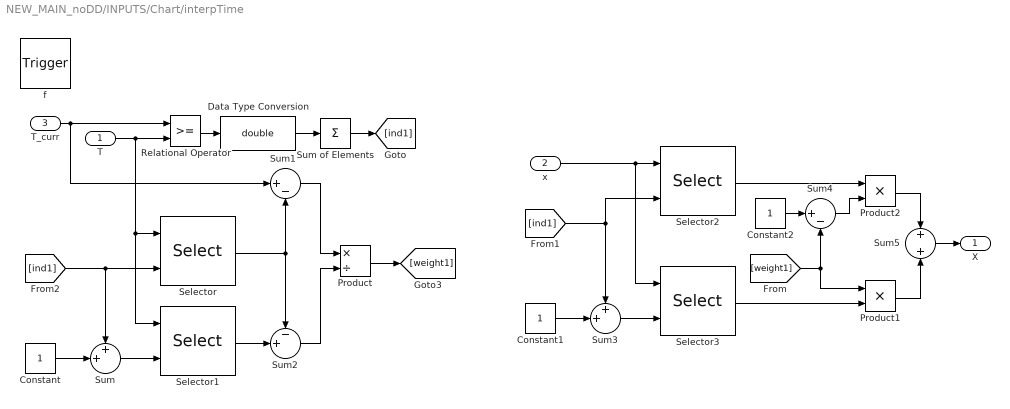
== system NEW_MAIN_noDD/INPUTS/Chart/interpTime ==
  T : Inport  OutDataTypeStr=double  PortDimensions=1
  x : Inport  Port=2  OutDataTypeStr=double  PortDimensions=1
  T_curr : Inport  Port=3  OutDataTypeStr=double  PortDimensions=1
  f : TriggerPort  TriggerType=function-call  VariantControl=(inherit)
      settings: CopyFcn=Stateflow.SLINSF.SimulinkMan.removeBlockPreDeleteFcn  PreDeleteFcn=Stateflow.SLINSF.SimulinkMan.unsafePredeleteFcn
  Constant : Constant
  Constant1 : Constant
  Constant2 : Constant
  Data Type Conversion : DataTypeConversion  OutDataTypeStr=double
  Product : Product  Inputs=*/
  Product1 : Product
  Product2 : Product
  Relational Operator : RelationalOperator  OutDataTypeStr=boolean  RndMeth=Simplest
  Selector{,1..3} (4 alike) : Selector  InputPortWidth=3  IndexOptions=Index vector (port)  Indices=[1 2 3]  OutputSizes=1
  Sum : Sum  Inputs=++|
  Sum of Elements : Sum  Inputs=+
  Sum1 : Sum  Inputs=|+-
  Sum2 : Sum  Inputs=-+|
  Sum3 : Sum  Inputs=++|
  Sum4 : Sum  Inputs=|+-
  Sum5 : Sum
  X : Outport
  wires:
  Relational Operator/1 -> Data Type Conversion/1
  Data Type Conversion/1 -> Sum of Elements/1
  Sum of Elements/1 -> [ind1]
  T/1 -> Selector1/1, Selector/1, Relational Operator/2
  [ind1] -> Sum/1, Selector/2
  Sum/1 -> Selector1/2
  Constant/1 -> Sum/2
  T_curr/1 -> Sum1/1, Relational Operator/1
  Selector/1 -> Sum1/2, Sum2/1
  Selector1/1 -> Sum2/2
  Sum1/1 -> Product/1
  Sum2/1 -> Product/2
  Product/1 -> [weight1]
  Sum3/1 -> Selector3/2
  Constant1/1 -> Sum3/2
  [ind1] -> Selector2/2, Sum3/1
  x/1 -> Selector3/1, Selector2/1
  Selector3/1 -> Product1/2
  [weight1] -> Product1/1, Sum4/2
  Constant2/1 -> Sum4/1
  Product1/1 -> Sum5/2
  Selector2/1 -> Product2/1
  Sum4/1 -> Product2/2
  Product2/1 -> Sum5/1
  Sum5/1 -> X/1

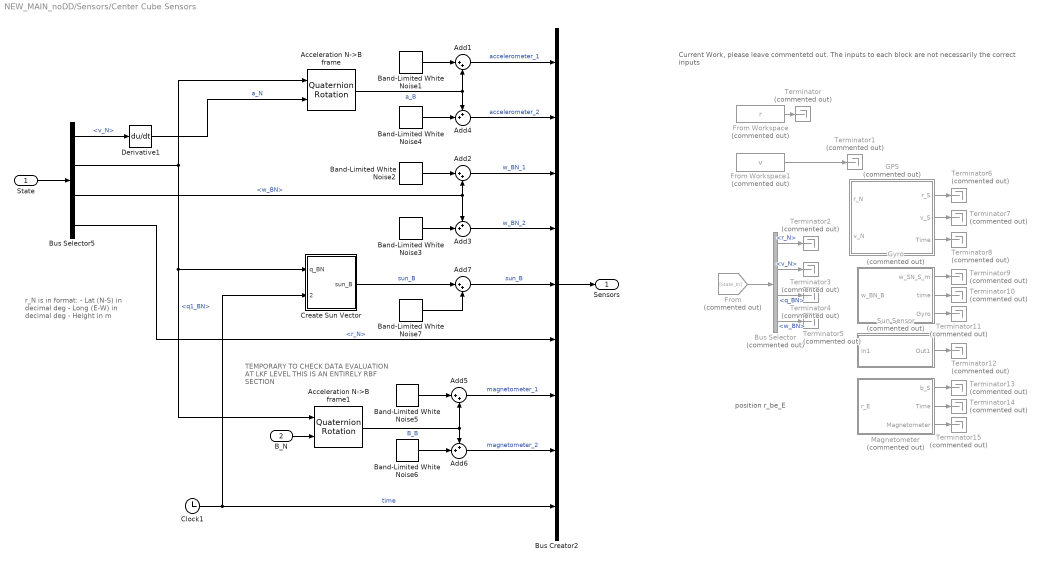
== system NEW_MAIN_noDD/Sensors/Center Cube Sensors ==
  note: Current Work, please leave commentetd out.
      | The inputs to each block are not necessarily
      | the correct inputs
  note: position r_be_E
  note: TEMPORARY TO CHECK DATA EVALUATION AT LKF LEVEL
      | THIS IS AN ENTIRELY RBF SECTION
  note: r_N is in format:
      | - Lat (N-S) in decimal deg
      | - Long (E-W) in decimal deg
      | - Height in m
  State : Inport
  B_N : Inport  Port=2
  Acceleration N->B frame : aerolibutil/Quaternion Rotation
  Acceleration N->B frame1 : aerolibutil/Quaternion Rotation
  Add{1..2,5,7} (4 alike) : Sum  Inputs=|++
  Add3 : Sum  Inputs=++|
  Add4 : Sum  Inputs=++|
  Add6 : Sum  Inputs=++|
  Band-Limited White Noise{1..7} (7 alike) : simulink/Sources/Band-Limited White Noise  Cov=[0.1]  Ts=1/freq  seed=[23341]
  Bus Creator2 : BusCreator  Inputs=9
  Bus Selector : BusSelector  Commented=on  OutputSignals=r_N,v_N,q_BN,w_BN
  Bus Selector5 : BusSelector  OutputSignals=v_N,q1_BN,w_BN,r_N
  Clock1 : Clock
  Create Sun Vector : Subsystem  AncestorBlock=SimMainLibrary/SideCubeSensors/Create Sun Vector  mask(Sun Vector){}
      mask help: This blocks takes the quaternion and GPS time, and calculates the unit vector pointing towards the sun. (Note: this vector can be relative to the position of the Earth or the position of the satellite, because the difference is negligible in relative magnitude.)
  Derivative1 : Derivative  CoefficientInTFapproximation=.01
  From : From  Commented=on  GotoTag=State_In
  From Workspace : FromWorkspace  Commented=on  VariableName=r  SampleTime=0
  From Workspace1 : FromWorkspace  Commented=on  VariableName=v  SampleTime=0
  GPS : Subsystem  Commented=on
  Gyro : Subsystem  Commented=on
  Magnetometer : Subsystem  Commented=on
  Sun Sensor : Subsystem  Commented=on
  Terminator{,1..15} (16 alike) : Terminator  Commented=on
  Sensors : Outport
  wires:
  Bus Selector5/4 -> Bus Creator2/6  "<r_N>"
  Add1/1 -> Bus Creator2/1  "accelerometer_1"
  Bus Selector5/1 -> Derivative1/1  "<v_N>"
  Band-Limited White Noise1/1 -> Add1/1
  Acceleration N->B frame/1 -> Add4/1, Add1/2  "a_B"
  Add4/1 -> Bus Creator2/2  "accelerometer_2"
  State/1 -> Bus Selector5/1
  Bus Creator2/1 -> Sensors/1
  Add7/1 -> Bus Creator2/5  "sun_B"
  Clock1/1 -> Create Sun Vector/2(GPS time), Bus Creator2/9  "time"
  Add3/1 -> Bus Creator2/4  "w_BN_2"
  Add2/1 -> Bus Creator2/3  "w_BN_1"
  Add6/1 -> Bus Creator2/8  "magnetometer_2"
  Add5/1 -> Bus Creator2/7  "magnetometer_1"
  Bus Selector5/2 -> Acceleration N->B frame1/1, Create Sun Vector/1(q_BN), Acceleration N->B frame/1  "<q1_BN>"
  From/1 -> Bus Selector/1
  From Workspace1/1 -> Terminator1/1
  From Workspace/1 -> Terminator/1
  Derivative1/1 -> Acceleration N->B frame/2  "a_N"
  Band-Limited White Noise4/1 -> Add4/2
  Band-Limited White Noise2/1 -> Add2/1
  Band-Limited White Noise3/1 -> Add3/2
  Bus Selector5/3 -> Add3/1, Add2/2  "<w_BN>"
  Create Sun Vector/1(sun_B) -> Add7/1  "sun_B"
  Band-Limited White Noise7/1 -> Add7/2
  Band-Limited White Noise6/1 -> Add6/2
  Band-Limited White Noise5/1 -> Add5/1
  Acceleration N->B frame1/1 -> Add6/1, Add5/2  "B_B"
  Bus Selector/1 -> Terminator2/1  "<r_N>"
  Bus Selector/2 -> Terminator3/1  "<v_N>"
  Bus Selector/3 -> Terminator4/1  "<q_BN>"
  Bus Selector/4 -> Terminator5/1  "<w_BN>"
  GPS/1(r_S) -> Terminator6/1
  GPS/2(v_S) -> Terminator7/1
  GPS/3(Time) -> Terminator8/1
  Gyro/1(w_SN_S_m) -> Terminator9/1
  Gyro/2(time) -> Terminator10/1
  Gyro/3(Gyro) -> Terminator11/1
  Sun Sensor/1(Out1) -> Terminator12/1
  Magnetometer/1(b_S) -> Terminator13/1
  Magnetometer/2(Time) -> Terminator14/1
  Magnetometer/3(Magnetometer) -> Terminator15/1
  B_N/1 -> Acceleration N->B frame1/2

== system NEW_MAIN_noDD/Sensors/EndSat Sensor1 ==
  note: Add Sensor Noise
  State : Inport
  B_N : Inport  Port=2
  Acceleration N->B frame : aerolibutil/Quaternion Rotation
  Add{1..2,4,6} (4 alike) : Sum  Inputs=|++
  Add3 : Sum  Inputs=++|
  Add5 : Sum  Inputs=++|
  Add8 : Sum  Inputs=++|
  Band-Limited White Noise{1..7} (7 alike) : simulink/Sources/Band-Limited White Noise  Cov=[0.1]  Ts=1/freq  seed=[23341]
  Bus Creator2 : BusCreator  Inputs=7
  Bus Selector5 : BusSelector  OutputSignals=v_N,q1_BN,w_BN,r_N
  Clock : Clock
  Create Sun Vector : SimMainLibrary/SideCubeSensors/Create Sun Vector
      settings: SourceProductName=CUGravity Library
  Magnetic Field Vector N->B frame : aerolibutil/Quaternion Rotation
  vel to acc : Derivative  CoefficientInTFapproximation=.01
  Sensors : Outport
  wires:
  Bus Selector5/4 -> Create Sun Vector/2  "<r_N>"
  Add8/1 -> Bus Creator2/2  "accelerometer_2"
  Band-Limited White Noise6/1 -> Add5/2
  Band-Limited White Noise5/1 -> Add4/1
  State/1 -> Bus Selector5/1
  Bus Selector5/1 -> vel to acc/1  "<v_N>"
  Band-Limited White Noise1/1 -> Add1/1
  Add1/1 -> Bus Creator2/1  "accelerometer_1"
  Add4/1 -> Bus Creator2/3  "magnetometer_1"
  Magnetic Field Vector N->B frame/1 -> Add5/1, Add4/2  "B_B"
  Bus Creator2/1 -> Sensors/1
  Bus Selector5/2 -> Create Sun Vector/1, Magnetic Field Vector N->B frame/1, Acceleration N->B frame/1  "<q1_BN>"
  Bus Selector5/3 -> Add2/2, Add3/1  "<w_BN>"
  Band-Limited White Noise4/1 -> Add8/2
  Add3/1 -> Bus Creator2/6  "w_BN_2"
  Add5/1 -> Bus Creator2/4  "magnetometer_2"
  Add2/1 -> Bus Creator2/5  "w_BN_1"
  Add6/1 -> Bus Creator2/7  "sun_B"
  Band-Limited White Noise7/1 -> Add6/2
  Create Sun Vector/1 -> Add6/1
  Band-Limited White Noise2/1 -> Add2/1
  Band-Limited White Noise3/1 -> Add3/2
  Acceleration N->B frame/1 -> Add1/2, Add8/1  "a_B"
  vel to acc/1 -> Acceleration N->B frame/2  "a_N"
  B_N/1 -> Magnetic Field Vector N->B frame/2
  Clock/1 -> Create Sun Vector/3

== system NEW_MAIN_noDD/Sensors/EndSat Sensor2 ==
  note: Things to Check:
      | Make sure that q1_BN is quaternion of B relative to N, otherwise rotation may be in the wrong direction.
      | Need to test the calculation to find the sun vector in the B frame.
  note: Add Sensor Noise
  State : Inport
  B_N : Inport  Port=2
  Acceleration N->B frame : aerolibutil/Quaternion Rotation
  Add{1..2,4,6} (4 alike) : Sum  Inputs=|++
  Add3 : Sum  Inputs=++|
  Add5 : Sum  Inputs=++|
  Add8 : Sum  Inputs=++|
  Band-Limited White Noise{1..7} (7 alike) : simulink/Sources/Band-Limited White Noise  Cov=[0.1]  Ts=1/freq  seed=[23341]
  Bus Creator2 : BusCreator  Inputs=7
  Bus Selector5 : BusSelector  OutputSignals=v_N,q1_BN,w_BN,r_N
  Clock : Clock
  Create Sun Vector : SimMainLibrary/SideCubeSensors/Create Sun Vector
      settings: SourceProductName=CUGravity Library
  Magnetic Field Vector N->B frame : aerolibutil/Quaternion Rotation
  vel to acc : Derivative  CoefficientInTFapproximation=.01
  Sensors : Outport
  wires:
  Bus Selector5/4 -> Create Sun Vector/2  "<r_N>"
  Add8/1 -> Bus Creator2/2  "accelerometer_2"
  Band-Limited White Noise6/1 -> Add5/2
  Band-Limited White Noise5/1 -> Add4/1
  State/1 -> Bus Selector5/1
  Bus Selector5/1 -> vel to acc/1  "<v_N>"
  Band-Limited White Noise1/1 -> Add1/1
  Add1/1 -> Bus Creator2/1  "accelerometer_1"
  Add4/1 -> Bus Creator2/3  "magnetometer_1"
  Magnetic Field Vector N->B frame/1 -> Add5/1, Add4/2  "B_B"
  Bus Creator2/1 -> Sensors/1
  Bus Selector5/2 -> Create Sun Vector/1, Magnetic Field Vector N->B frame/1, Acceleration N->B frame/1  "<q1_BN>"
  Bus Selector5/3 -> Add2/2, Add3/1  "<w_BN>"
  Band-Limited White Noise4/1 -> Add8/2
  Add3/1 -> Bus Creator2/6  "w_BN_2"
  Add5/1 -> Bus Creator2/4  "magnetometer_2"
  Add2/1 -> Bus Creator2/5  "w_BN_1"
  Add6/1 -> Bus Creator2/7  "sun_B"
  Band-Limited White Noise7/1 -> Add6/2
  Create Sun Vector/1 -> Add6/1
  Band-Limited White Noise2/1 -> Add2/1
  Band-Limited White Noise3/1 -> Add3/2
  Acceleration N->B frame/1 -> Add1/2, Add8/1  "a_B"
  vel to acc/1 -> Acceleration N->B frame/2  "a_N"
  B_N/1 -> Magnetic Field Vector N->B frame/2
  Clock/1 -> Create Sun Vector/3

== system NEW_MAIN_noDD/Flight Computers/Center Cube Controller/SafeMode ==
  GrndCmds : Inport
  Safe Mode In : Inport  Port=2
  Pwbrd : Inport  Port=3
  "EKFhs " : Inport  Port=4
  EstState : Inport  Port=5
  B_N : Inport  Port=6
  Bus Selector : BusSelector  OutputSignals=GrdOM,GrdSEPC
  Bus Selector2 : BusSelector  OutputSignals=ADCSAks,PwbrdCmmds.PbOpMode,PwbrdCmmds.PbSepCmmd
  Clock1 : Clock
  Gain : Gain  Gain=[1;1;1;1]
  STATUS_MODE_DETERMINATION : Stateflow chart  TreatAsAtomicUnit=on  mask(ACS State Machine){KpS=epsilon_UD_slew^2*.01, KdS=epsilon_UD_slew*.3, KpSU=epsilon_UD_spinUp^2*.05, KdSU=epsilon_UD_spinUp*0.025}
      mask prompts: KpS "Slew Proportional Gain"; KdS "Slew Derivative Gain"; KpSU "Spin Up Proportional Gain"; KdSU "Spin Up Derivative Gain"
      mask help:
      | The is the main state machine and safe mode filter for the ADCS block.
      |
      | The ADCS Status Chart checks the incoming Ak signals to ensure all components (sensors and actuators) are working properly. If not, this chart notifies the State Machine.
      |
      | The State Machine determines the mode switching logic based off of a thrown Safe Mode signal and possible component level issues.
      |
      | The outputs are:
      | 1. SafeOpMode - operating mode of the Flight Computer based on State Machine decision.
      | 2. Updated State Variables
      | 3. SafeMode_Out - true is Safe Mode is still required, false if override command has been received from powerboard
      |
      | Resources:
      | 1. ADCS Design (Fall 2016)
  TORQUE_MANAGEMENT : Subsystem
  Terminator1 : Terminator
  Terminator3 : Terminator
  SafedOpMode : Outport
  SafedSeperationBurn : Outport  Port=2
  PwbMEX : Outport  Port=3
  T_N : Outport  Port=4
  Safed Att. State : Outport  Port=5
  Safe Mode Out : Outport  Port=6
  wires:
  Bus Selector/1 -> STATUS_MODE_DETERMINATION/7(OpMode)  "<GrdOM>"
  GrndCmds/1 -> Bus Selector/1
  Safe Mode In/1 -> STATUS_MODE_DETERMINATION/5(SafeMode_In)  "SafeMode_In"
  Bus Selector/2 -> Gain/1, STATUS_MODE_DETERMINATION/8(SepCmd)  "<GrdSEPC>"
  Pwbrd/1 -> Bus Selector2/1
  Bus Selector2/1 -> STATUS_MODE_DETERMINATION/1(Ak)  "<ADCSAks>"
  Gain/1 -> SafedSeperationBurn/1
  Clock1/1 -> STATUS_MODE_DETERMINATION/4(t)
  STATUS_MODE_DETERMINATION/6(SafeMode_Out) -> Safe Mode Out/1
  STATUS_MODE_DETERMINATION/7(PwbMEX) -> PwbMEX/1
  "EKFhs "/1 -> STATUS_MODE_DETERMINATION/6(EKFHs)  "EKFhs"
  Bus Selector2/2 -> STATUS_MODE_DETERMINATION/2(PbOpMode)  "<PbOpMode>"
  STATUS_MODE_DETERMINATION/8(SafedOpMode) -> SafedOpMode/1
  Bus Selector2/3 -> STATUS_MODE_DETERMINATION/3(SEPC)  "<PbSepCmmd>"
  STATUS_MODE_DETERMINATION/1(MODE) -> TORQUE_MANAGEMENT/1(MODE)
  STATUS_MODE_DETERMINATION/2(KP) -> TORQUE_MANAGEMENT/2(Kp)
  STATUS_MODE_DETERMINATION/3(KD) -> TORQUE_MANAGEMENT/3(Kd)
  B_N/1 -> TORQUE_MANAGEMENT/5(B_N)
  TORQUE_MANAGEMENT/1(T_N) -> T_N/1
  TORQUE_MANAGEMENT/2(Safed Att. State) -> Safed Att. State/1
  EstState/1 -> TORQUE_MANAGEMENT/4(EstState)
  STATUS_MODE_DETERMINATION/4(Actuator_Health) -> Terminator3/1
  STATUS_MODE_DETERMINATION/5(IMU_Health) -> Terminator1/1

== system NEW_MAIN_noDD/Flight Computers/Center Cube Controller/Torque Coil Management ==
  note: Why does torque coils suddenly become PWM?
  B_N : Inport
  torque_cmd_N : Inport  Port=2
  q : Inport  Port=3
  Calculate Coil Torque and Current : Subsystem
  Constant4 : Constant  Value=sat2CoilArea.*sat2n.*currentMax_B
  Magnetic Moment Unit Vector : Subsystem
  Magnetic Moment Vector : Subsystem
  Product2 : Product
  Quaternion Rotation : aerolibutil/Quaternion Rotation
  Reduce Wasted Effort : Subsystem
  Saturation : Saturate  Commented=on  UpperLimit=magMomentMax_B(2:3)  LowerLimit=-magMomentMax_B(2:3)
  Selector : Selector  InputPortWidth=3  IndexOptions=Index vector (dialog)  Indices=[2 3]  OutputSizes=1
  Vector Saturation1 : SimMainLibrary/Vector Saturation
      settings: SourceProductName=CUGravity Library
  torque : Constant  Commented=on  Value=[0;1;-1]
  torque_coils : Outport
  CenterCube_PWM_cmds : Outport  Port=2
  wires:
  Constant4/1 -> Selector/1
  B_N/1 -> Calculate Coil Torque and Current/4(B_N), Quaternion Rotation/2
  q/1 -> Quaternion Rotation/1, Calculate Coil Torque and Current/3(q), Magnetic Moment Unit Vector/2(q)
  Reduce Wasted Effort/1(mu_sat_B1) -> Calculate Coil Torque and Current/2(mu_B23)  "mu_B23"
  Vector Saturation1/1 -> Reduce Wasted Effort/2(mu_sat_B)  "mu_sat_B"
  torque_cmd_N/1 -> Magnetic Moment Vector/2(torque_cmd_N), Calculate Coil Torque and Current/1(torque_cmd_N), Magnetic Moment Unit Vector/1(torque_cmd_N)  "torque_cmd_N"
  Magnetic Moment Unit Vector/1(muHat_B) -> Magnetic Moment Vector/1(muHat_B), Reduce Wasted Effort/1(muHat_B)
  Quaternion Rotation/1 -> Reduce Wasted Effort/3(B_B), Magnetic Moment Vector/3(B_B)  "B_B"
  Product2/1 -> torque_coils/1
  Magnetic Moment Vector/1(mu_raw_B) -> Vector Saturation1/1  "mu_raw_B"
  Calculate Coil Torque and Current/1(torque_N) -> Product2/1
  Calculate Coil Torque and Current/2(Sign_B & mu) -> Product2/2
  Calculate Coil Torque and Current/3(coils_I) -> CenterCube_PWM_cmds/1
  Selector/1 -> Vector Saturation1/2

== system NEW_MAIN_noDD/Flight Computers/CenterCube EKF/Kalman Gain and Estamated State Computation ==
  P_kp : Inport
  x_kp : Inport  Port=2
  Y : Inport  Port=3
  " LU Inverse" : dspinverses/ LU Inverse
      settings: SourceProductName=DSP System Toolbox
  Add1 : Sum
  Add2 : Sum
  Add3 : Sum  Inputs=-+
  H : Constant  Value=H
  H1 : Constant  Value=H
  Math Function : Math  Operator=transpose  SaturateOnIntegerOverflow=on
  Product{,1,3..4,6} (5 alike) : Product  Multiplication=Matrix(*)
  Product2 : Product
  R : Constant  Value=R
  K : Outport
  x_k : Outport  Port=2
  wires:
  H/1 -> Product3/1, Product1/2, Math Function/1
  " LU Inverse"/1 -> Product/2
  Product1/1 -> Product/1
  Math Function/1 -> Product4/2
  Product/1 -> Product2/1, K/1  "Kalman Gain K"
  x_kp/1 -> Add2/1, Product6/2
  Y/1 -> Add3/2
  R/1 -> Add1/2
  Product4/1 -> Add1/1
  Add1/1 -> " LU Inverse"/1
  Product3/1 -> Product4/1
  H1/1 -> Product6/1
  Product6/1 -> Add3/1
  P_kp/1 -> Product3/2, Product1/1
  Add2/1 -> x_k/1
  Add3/1 -> Product2/2
  Product2/1 -> Add2/2
